simulink model "ACC_Model"  (Simulink 7.6)
settings: Solver=ode5  StartTime=0.0  StopTime=inf  FixedStep=1/100  RelTol=1e-3
undefined symbols (not defined in the file or in its folder): DiscIntNeverNeededParam
libraries: simulink x21, simulink_extras x6
(part 2 of 4)

== system ACC_Model/ACC_System/TIS2 Straight Road ==
  note: === TIS2 Straight Road block ===
      |
      |  - interpretes information provided from the second TIS sensor,
      |  - computes HeadWay Time (HWT) for object on the lane in front of the EGO car,
      |  - determines if detected objects is potentially dengerous,
      |  - outputs distance to the following car, computes its velocity and safe distance to be kept.
  EGO_velocity [m/s] : Inport
  TIS2_range [m] : Inport  Port=2  PortDimensions=TISdet(2)
  TIS2_rangedot [m/s] : Inport  Port=3  PortDimensions=TISdet(2)
  TIS2_theta [deg] : Inport  Port=4  PortDimensions=TISdet(2)
  HWT_dem [s] : Inport  Port=5
  Standstill [m] : Inport  Port=6
  HWT_dem [s]1 : InportShadow  Port=5
  Hold : Subsystem
  TIS2 Closest Object : Subsystem
  TIS2 HWT Computing : Subsystem
  TIS2 HWT Computing2 : Subsystem
  TIS2 HWT Flag : Subsystem
  TIS2 Lead Car Longitudinal Velocity : Subsystem
  TIS2 Objects On Lane : Subsystem
  TIS2 Sorting Fun : Subsystem
  TIS2_closest_object_search : Stateflow chart  TreatAsAtomicUnit=on
  HWT_flag : Outport
  TIS2 Lead distance [m] : Outport  Port=2
  TIS2 Safe_distance [m] : Outport  Port=3
  TIS2_HWT_straight : Outport  Port=4
  TIS2 Lead velocity [m/s] : Outport  Port=5
  index : Outport  Port=6
  wires:
  TIS2 Lead Car Longitudinal Velocity/1(Safe distance [m]) -> TIS2 Safe_distance [m]/1
  HWT_dem [s]/1 -> TIS2 Lead Car Longitudinal Velocity/1(HWT_dem (s)), TIS2 HWT Flag/2(HWT_dem [s])
  TIS2 Closest Object/1(rangedot [m/s]) -> TIS2 Lead Car Longitudinal Velocity/2(TIS2 Rangedot [m/s])
  TIS2 Closest Object/2(distance [m/s]) -> TIS2 Lead distance [m]/1, TIS2 HWT Computing2/1(Distance [m]), TIS2 HWT Flag/1(Distance closest [m])
  EGO_velocity [m/s]/1 -> TIS2 Lead Car Longitudinal Velocity/3(EGO Velocity [m/s]), TIS2 HWT Computing2/2(Velocity [m/s]), TIS2 HWT Computing/3(Velocity [m/s])
  TIS2 HWT Computing/1(HWT [s]) -> TIS2 HWT Flag/3(HWT [s])
  TIS2_closest_object_search/1(index) -> TIS2 Closest Object/3(index), index/1
  TIS2 Sorting Fun/3(TIS2_THETA [rad]) -> TIS2 Objects On Lane/3(TIS2_theta [rad])
  TIS2 Sorting Fun/2(TIS2_RANGEDOT [m/s]) -> TIS2 Objects On Lane/2(TIS2_rangedot [m/s])
  TIS2 Sorting Fun/1(TIS2_RANGE [m]) -> TIS2 Objects On Lane/1(TIS2_range [m])
  TIS2_theta [deg]/1 -> TIS2 Sorting Fun/3(TIS2theta [deg])
  TIS2_rangedot [m/s]/1 -> TIS2 Sorting Fun/2(TIS2rangedot [m/s])
  TIS2_range [m]/1 -> TIS2 Sorting Fun/1(TIS2range [m])
  Standstill [m]/1 -> TIS2 Lead Car Longitudinal Velocity/4(Standstill [m]), TIS2 HWT Flag/4(Standstill distance)
  TIS2 Objects On Lane/1(TIS2_RANGEDOT [m/s]) -> TIS2 Closest Object/1(TIS2_rangedot [m/s])
  TIS2 Lead Car Longitudinal Velocity/2(Lead velocity [m/s]) -> TIS2 Lead velocity [m/s]/1, Hold/2(lead_vel_in)
  TIS2 HWT Computing2/1(HWT [s]) -> TIS2_HWT_straight/1
  TIS2 HWT Flag/1(HWT_flag) -> Hold/1(HWTflagIN)
  Hold/1(HWT_flag) -> HWT_flag/1
  HWT_dem [s]1/1 -> TIS2 HWT Computing/2(HWT demanded)
  TIS2 Objects On Lane/2(TIS2_Distance [m]) -> TIS2 Closest Object/2(TIS2_distance [m]), TIS2_closest_object_search/1(distance), TIS2 HWT Computing/1(Distance [m])

== system ACC_Model/ACC_System/Display/If Action Subsystem ==
  note: === Display Module ===
      |
      |  - calls a GUI, which is updated at each step time,
      |  - Inputs for 'DISPLAY' block (msfcn_PlotSpeed):
      |    1 - RPM
      |    2 - EGO Velocity [kph]
      |    3 - Brake Pressure [bar]
      |    4 - Throttle [%]
      |    5 - ACC Flag
      |    6 - HWT converted
      |    7 - Lead car velocity [m/s]
      |
      |  - Output from DISPLAY block (msfcn_ACC_PlotSpeed function):
      |    1 - ACC system manual switch {0 - system off, 1 - system on}
  RPM1 : Inport
  EGO Velocity [m/s]1 : Inport  Port=2
  Brake_Pressure_[bar]1 : Inport  Port=3
  HWT_%1 : Inport  Port=4
  ACC_flag1 : Inport  Port=5
  Lead_car_velocity_[m/s]1 : Inport  Port=6
  Throttle_[%]1 : Inport  Port=7
  Action Port : ActionPort  PropagateVarSize=During execution  ActionType=then
  Brake Pressure [bar] : Gain  Gain=100/BrakePressureMax
  Brake Pressure [bar]1 : Gain  Gain=3.6
  DISPLAY : M-S-Function  FunctionName=msfcn_ACC_PlotSpeed  Parameters=DisplayFreq DisplaySwitch
      mask Display:
      | port_label('input',1,'RPM');
      | port_label('input',2,'EGO Velocity [km/h]');
      | port_label('input',3,'Brake Pressure [bar]');
      | port_label('input',4,'Throttle [%]');
      | port_label('input',5,'ACC Flag');
      | port_label('input',6,'HWT/HWT_dem-1 [%]');
      | port_label('input',7,'Lead car velocity [m/s]');
      | 
      | port_label('output',1,'System On/Off');
  Gain : Gain  OutDataTypeStr=double
  Rounding Function{,1..4,6} (6 alike) : Rounding  Operator=round
  m/s_kph1 : Gain  Gain=3.6
  "GUI_System ON {1} / OFF {0}1" : Outport  InitialOutput=1
  wires:
  Rounding Function/1 -> DISPLAY/1
  Rounding Function1/1 -> DISPLAY/2
  Rounding Function2/1 -> DISPLAY/3
  Rounding Function3/1 -> DISPLAY/4
  Brake Pressure [bar]/1 -> Rounding Function2/1
  Brake_Pressure_[bar]1/1 -> Brake Pressure [bar]/1
  Throttle_[%]1/1 -> Rounding Function3/1
  RPM1/1 -> Rounding Function/1
  m/s_kph1/1 -> Rounding Function4/1
  Rounding Function4/1 -> DISPLAY/7
  Rounding Function6/1 -> DISPLAY/5
  Gain/1 -> Rounding Function6/1
  EGO Velocity [m/s]1/1 -> Brake Pressure [bar]1/1
  ACC_flag1/1 -> Gain/1
  Lead_car_velocity_[m/s]1/1 -> m/s_kph1/1
  DISPLAY/1 -> "GUI_System ON {1} / OFF {0}1"/1
  HWT_%1/1 -> DISPLAY/6
  Brake Pressure [bar]1/1 -> Rounding Function1/1

== system ACC_Model/ACC_System/Display/If Action Subsystem1 ==
  Action Port : ActionPort  PropagateVarSize=During execution  ActionType=else
  Constant : Constant
  Out1 : Outport  InitialOutput=1
  wires:
  Constant/1 -> Out1/1

== system ACC_Model/ACC_System/Limitations1/cond ==
  In1 : Inport
  Integer Delay : simulink/Discrete/Integer Delay  NumDelays=1/Tsensor  InputProcessing=Inherited  vinit=0.0  samptime=Tsensor
  Logical Operator2 : Logic  Operator=NOT  AllPortsSameDT=off  OutDataTypeStr=boolean
  Logical Operator3 : Logic  Operator=OR  AllPortsSameDT=off  OutDataTypeStr=boolean
  Out1 : Outport
  wires:
  Logical Operator2/1 -> Logical Operator3/1, Integer Delay/1
  Integer Delay/1 -> Logical Operator3/2
  In1/1 -> Logical Operator2/1
  Logical Operator3/1 -> Out1/1

== system ACC_Model/ACC_System/Limitations2/cond1 ==
  In1 : Inport
  Integer Delay : simulink/Discrete/Integer Delay  NumDelays=1/Tsensor  InputProcessing=Inherited  vinit=0.0  samptime=Tsensor
  Logical Operator3 : Logic  Operator=OR  AllPortsSameDT=off  OutDataTypeStr=boolean
  Out1 : Outport
  wires:
  Integer Delay/1 -> Logical Operator3/2
  In1/1 -> Logical Operator3/1, Integer Delay/1
  Logical Operator3/1 -> Out1/1

== system ACC_Model/ACC_System/Radar/Radar ==
  TIS1 Range : Inport
  TIS1 Theta : Inport  Port=2
  TIS2 Range : Inport  Port=3
  TIS2 Theta : Inport  Port=4
  TIS1_index : Inport  Port=5
  TIS2_index : Inport  Port=6
  TIS1_HWT_% : Inport  Port=7
  TIS2_HWT_% : Inport  Port=8
  System switch : Inport  Port=9
  Enable : EnablePort  PropagateVarSize=During execution
  Level-2 M-file S-Function : M-S-Function  FunctionName=msfcn_ACC_radar_graph  Parameters=RadarFreq TISdet TISMaxRange TISMaxTheta RadarSwitch
  Logical Operator : Logic  AllPortsSameDT=off  OutDataTypeStr=boolean
  Logical Operator1 : Logic  AllPortsSameDT=off  OutDataTypeStr=boolean
  Product1 : Product  RndMeth=Zero
  Product2 : Product  RndMeth=Zero
  wires:
  TIS1 Range/1 -> Level-2 M-file S-Function/1
  TIS1 Theta/1 -> Level-2 M-file S-Function/2
  TIS2 Range/1 -> Level-2 M-file S-Function/3
  TIS2 Theta/1 -> Level-2 M-file S-Function/4
  TIS1_HWT_%/1 -> Logical Operator/1
  TIS2_HWT_%/1 -> Logical Operator1/1
  Logical Operator/1 -> Level-2 M-file S-Function/7
  Logical Operator1/1 -> Level-2 M-file S-Function/8
  System switch/1 -> Logical Operator1/2, Logical Operator/2, Product2/2, Product1/2
  Product2/1 -> Level-2 M-file S-Function/6
  Product1/1 -> Level-2 M-file S-Function/5
  TIS1_index/1 -> Product1/1
  TIS2_index/1 -> Product2/1

== system ACC_Model/ACC_System/TIS1 ACC action/If Action Subsystem ==
  rd : Inport
  e : Inport  Port=2
  Vp : Inport  Port=3
  EGO distance : Inport  Port=4
  HWT dem : Inport  Port=5
  th in : Inport  Port=6
  Action Port : ActionPort  PropagateVarSize=During execution  ActionType=then
  If : If  IfExpression=u1 <= 0  SampleTime=Tsensor
  If Action Subsystem : Subsystem  TreatAsAtomicUnit=on
  If Action Subsystem1 : Subsystem  TreatAsAtomicUnit=on
  Merge : Merge
  Merge1 : Merge
  Rate Limiter : RateLimiter  RisingSlewLimit=BrakeMax*1e3  FallingSlewLimit=-BrakeMax*1e3  SampleTimeMode=inherited
  e1 : InportShadow  Port=2
  th in1 : InportShadow  Port=6
  dec : Outport  InitialOutput=0
  throttle : Outport  Port=2  InitialOutput=0
  wires:
  rd/1 -> If/1, If Action Subsystem1/1(rd)
  If/1 -> If Action Subsystem/Action
  If/2 -> If Action Subsystem1/Action
  e/1 -> If Action Subsystem/1(e)
  If Action Subsystem/1(brake) -> Merge/1
  If Action Subsystem1/1(dec) -> Merge/2
  If Action Subsystem/2(throttle) -> Merge1/1
  If Action Subsystem1/2(throttle) -> Merge1/2
  Merge/1 -> dec/1
  Merge1/1 -> Rate Limiter/1
  Vp/1 -> If Action Subsystem1/3(Vp)
  e1/1 -> If Action Subsystem1/2(e)
  EGO distance/1 -> If Action Subsystem1/4(EGO distance)
  HWT dem/1 -> If Action Subsystem1/5(HWT_dem)
  th in/1 -> If Action Subsystem/2(th_in)
  th in1/1 -> If Action Subsystem1/6(th_in)
  Rate Limiter/1 -> throttle/1

== system ACC_Model/ACC_System/TIS1 ACC action/If Action Subsystem1 ==
  rd : Inport
  e : Inport  Port=2
  Vp : Inport  Port=3
  EGO dis : Inport  Port=4
  HWT dem : Inport  Port=5
  Action Port : ActionPort  PropagateVarSize=During execution  ActionType=else
  If : If  IfExpression=u1 <= 0  SampleTime=Tsensor
  If Action Subsystem : Subsystem  TreatAsAtomicUnit=on
  If Action Subsystem1 : Subsystem  TreatAsAtomicUnit=on
  Merge : Merge
  Merge1 : Merge
  dec : Outport  InitialOutput=0
  throttle : Outport  Port=2  InitialOutput=0
  wires:
  rd/1 -> If/1, If Action Subsystem1/1(rd)
  If/1 -> If Action Subsystem/Action
  If/2 -> If Action Subsystem1/Action
  Vp/1 -> If Action Subsystem1/3(Vp)
  If Action Subsystem/1(dec) -> Merge/1
  If Action Subsystem1/2(throttle) -> Merge1/2
  Merge/1 -> dec/1
  Merge1/1 -> throttle/1
  If Action Subsystem1/1(dec) -> Merge/2
  If Action Subsystem/2(throttle) -> Merge1/1
  e/1 -> If Action Subsystem1/2(e)
  EGO dis/1 -> If Action Subsystem1/4(Ego distance)
  HWT dem/1 -> If Action Subsystem1/5(HWT dem)

== system ACC_Model/ACC_System/TIS1 Bend Road/Hold ==
  HWTflagIN : Inport
  lead_vel_in : Inport  Port=2
  HWTflagIN1 : InportShadow  Port=1
  If : If  IfExpression=u1 < 0.1  SampleTime=Tsensor
  If Action Subsystem : Subsystem  TreatAsAtomicUnit=on
  If Action Subsystem1 : Subsystem  TreatAsAtomicUnit=on
  Merge : Merge
  HWT_flag : Outport
  wires:
  lead_vel_in/1 -> If/1
  If/1 -> If Action Subsystem/Action
  If/2 -> If Action Subsystem1/Action
  If Action Subsystem/1(Out1) -> Merge/1
  If Action Subsystem1/1(Out1) -> Merge/2
  Merge/1 -> HWT_flag/1
  HWTflagIN/1 -> If Action Subsystem1/1(In1)
  HWTflagIN1/1 -> If Action Subsystem/1(In1)

== system ACC_Model/ACC_System/TIS1 Bend Road/Lead Car Longitudinal Velocity ==
  note: === TIS1 Lead Car Longitudinal Velocity block ===
      |
      |  - computes the leading car absolute velocity and safe distance between the EGO and leading car.
  HWT_dem (s) : Inport
  TIS1 Rangedot [m/s] : Inport  Port=2
  EGO Velocity [m/s] : Inport  Port=3
  Standstill [m] : Inport  Port=4
  theta [rad] : Inport  Port=5
  lambda [rad] : Inport  Port=6
  TIS1 Range [m] : Inport  Port=7
  Abs : Abs
  Add : Sum  Inputs=+-  RndMeth=Zero
  Add1 : Sum  Inputs=+-
  Constant : Constant  Value=0
  Divide : Product  Inputs=*/
  Divide2 : Product  Inputs=*/
  HWT_dem (s)1 : InportShadow  Port=1
  Product : Product  RndMeth=Zero
  Relational Operator : RelationalOperator  Operator=<=  OutDataTypeStr=boolean
  Switch : Switch  Criteria=u2 > Threshold
  Switch1 : Switch  Threshold=TISMaxRange(1)
  Trigonometric Function : Trigonometry  Operator=cos
  Safe distance [m] : Outport
  Lead velocity [m/s] : Outport  Port=2
  wires:
  Relational Operator/1 -> Switch/2
  Divide/1 -> Relational Operator/2
  HWT_dem (s)1/1 -> Divide/2
  Standstill [m]/1 -> Switch/1, Divide/1
  Switch/1 -> Safe distance [m]/1
  Product/1 -> Switch/3
  HWT_dem (s)/1 -> Product/2
  Add/1 -> Abs/1
  TIS1 Rangedot [m/s]/1 -> Divide2/1
  EGO Velocity [m/s]/1 -> Add/1
  lambda [rad]/1 -> Add1/1
  theta [rad]/1 -> Add1/2
  Add1/1 -> Trigonometric Function/1
  Trigonometric Function/1 -> Divide2/2
  Divide2/1 -> Add/2
  Abs/1 -> Product/1, Relational Operator/1, Switch1/3
  TIS1 Range [m]/1 -> Switch1/2
  Constant/1 -> Switch1/1
  Switch1/1 -> Lead velocity [m/s]/1

== system ACC_Model/ACC_System/TIS1 Bend Road/TIS1 Closest Object On Bend Road ==
  note: === TIS1 Closest Object block ===
      |
      |  - passing through data about potentially the most dangerous object driving on the bend road.
  index : Inport
  TIS1_range [m] : Inport  Port=2
  TIS1_rangedot [m] : Inport  Port=3
  TIS1_theta [rad] : Inport  Port=4
  TIS1_Distance [m] : Inport  Port=5
  TIS1_lambda [rad] : Inport  Port=6
  Constant2 : Constant  Value=TISMaxRange(1)
  Selector{1..3,6..7} (5 alike) : Selector  InputPortWidth=TISdet(1)  IndexOptions=Index vector (port)  Indices=[1 3]  OutputSizes=1
  Switch : Switch  Criteria=u2 ~= 0
  range [m] : Outport
  rangedot [m/s] : Outport  Port=2
  theta [rad] : Outport  Port=3
  Distance [m] : Outport  Port=4
  lambda [rad] : Outport  Port=5
  wires:
  TIS1_rangedot [m]/1 -> Selector2/1
  TIS1_range [m]/1 -> Selector1/1
  index/1 -> Selector1/2, Selector2/2, Selector3/2, Selector6/2, Selector7/2
  TIS1_theta [rad]/1 -> Selector3/1
  TIS1_Distance [m]/1 -> Selector6/1
  TIS1_lambda [rad]/1 -> Selector7/1
  Selector1/1 -> range [m]/1
  Selector2/1 -> rangedot [m/s]/1
  Selector3/1 -> theta [rad]/1
  Selector7/1 -> lambda [rad]/1
  Selector6/1 -> Switch/2, Switch/1
  Constant2/1 -> Switch/3
  Switch/1 -> Distance [m]/1

== system ACC_Model/ACC_System/TIS1 Bend Road/TIS1 HWT Computing ==
  note: === TIS1 HWT Computing block===
      |
      |  - computes HeadWay Time (HWT) as it is defined in ISO norms.
  Distance [m] : Inport
  Velocity [m/s] : Inport  Port=2
  If : If
  If Action Subsystem : Subsystem  TreatAsAtomicUnit=on
  If Action Subsystem1 : Subsystem  TreatAsAtomicUnit=on
  Merge : Merge
  HWT [s] : Outport
  wires:
  Velocity [m/s]/1 -> If/1, If Action Subsystem/2(Velocity [m/s])
  If/1 -> If Action Subsystem/Action
  If/2 -> If Action Subsystem1/Action
  If Action Subsystem/1(HWT [s]) -> Merge/1
  If Action Subsystem1/1(Out1) -> Merge/2
  Merge/1 -> HWT [s]/1
  Distance [m]/1 -> If Action Subsystem/1(Distance [m])

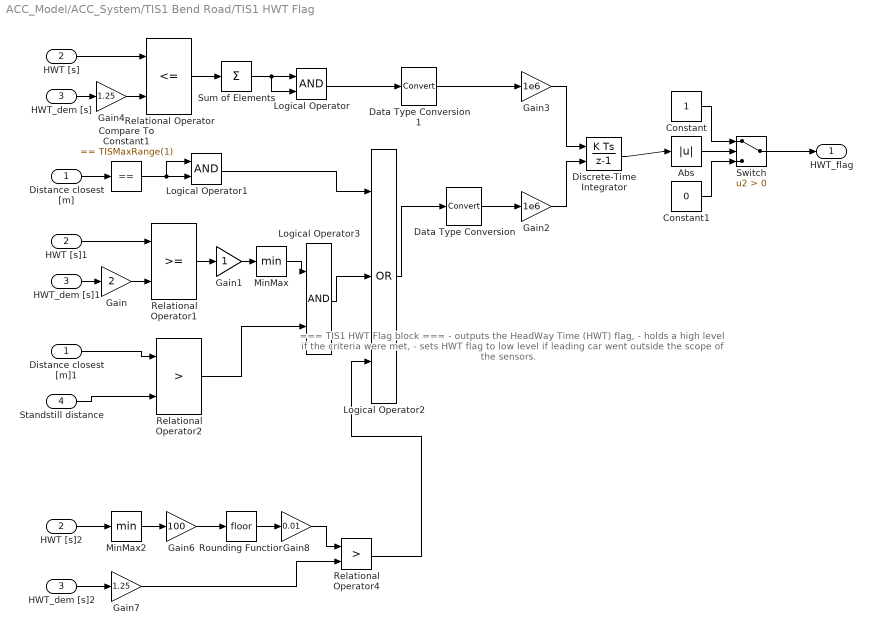
== system ACC_Model/ACC_System/TIS1 Bend Road/TIS1 HWT Flag ==
  note: === TIS1 HWT Flag block ===
      |
      |  - outputs the HeadWay Time (HWT) flag,
      |  - holds a high level if the criteria were met,
      |  - sets HWT flag to low level if leading car
      |    went outside the scope of the sensors.
  Distance closest [m] : Inport
  HWT [s] : Inport  Port=2
  HWT_dem [s] : Inport  Port=3
  Standstill distance : Inport  Port=4
  Abs : Abs
  Compare To Constant1 : simulink/Logic and Bit Operations/Compare To Constant  SystemSampleTime=-1  relop===  const=TISMaxRange(1)  LogicOutDataTypeMode=uint8
  Constant : Constant
  Constant1 : Constant  Value=0
  Data Type Conversion : DataTypeConversion
  Data Type Conversion1 : DataTypeConversion
  Discrete-Time Integrator : DiscreteIntegrator  ExternalReset=level  SampleTime=Tsensor  ICPrevOutput=DiscIntNeverNeededParam  ICPrevScaledInput=DiscIntNeverNeededParam
  Distance closest [m]1 : InportShadow  Port=1
  Gain : Gain  Gain=2
  Gain1 : Gain
  Gain2 : Gain  Gain=1e6  OutDataTypeStr=double
  Gain3 : Gain  Gain=1e6  OutDataTypeStr=double
  Gain4 : Gain  Gain=1.25
  Gain6 : Gain  Gain=100
  Gain7 : Gain  Gain=1.25
  Gain8 : Gain  Gain=0.01
  HWT [s]1 : InportShadow  Port=2
  HWT [s]2 : InportShadow  Port=2
  HWT_dem [s]1 : InportShadow  Port=3
  HWT_dem [s]2 : InportShadow  Port=3
  Logical Operator : Logic  AllPortsSameDT=off  OutDataTypeStr=boolean
  Logical Operator1 : Logic  AllPortsSameDT=off  OutDataTypeStr=boolean
  Logical Operator2 : Logic  Operator=OR  Inputs=3  AllPortsSameDT=off  OutDataTypeStr=boolean
  Logical Operator3 : Logic  AllPortsSameDT=off  OutDataTypeStr=boolean
  MinMax : MinMax
  MinMax2 : MinMax
  Relational Operator : RelationalOperator  Operator=<=  OutDataTypeStr=boolean
  Relational Operator1 : RelationalOperator  OutDataTypeStr=boolean
  Relational Operator2 : RelationalOperator  Operator=>  OutDataTypeStr=boolean
  Relational Operator4 : RelationalOperator  Operator=>  OutDataTypeStr=boolean
  Rounding Function : Rounding
  Sum of Elements : Sum  Inputs=+
  Switch : Switch  Criteria=u2 > Threshold
  HWT_flag : Outport
  wires:
  Logical Operator1/1 -> Logical Operator2/1
  Distance closest [m]/1 -> Compare To Constant1/1
  Logical Operator/1 -> Data Type Conversion1/1
  Sum of Elements/1 -> Logical Operator/2, Logical Operator/1
  Relational Operator/1 -> Sum of Elements/1
  HWT_dem [s]/1 -> Gain4/1
  HWT [s]/1 -> Relational Operator/1
  Compare To Constant1/1 -> Logical Operator1/2, Logical Operator1/1
  HWT [s]1/1 -> Relational Operator1/1
  Gain/1 -> Relational Operator1/2
  Relational Operator1/1 -> Gain1/1
  Gain1/1 -> MinMax/1
  Logical Operator2/1 -> Data Type Conversion/1
  HWT_dem [s]1/1 -> Gain/1
  Distance closest [m]1/1 -> Relational Operator2/1
  Standstill distance/1 -> Relational Operator2/2
  Relational Operator2/1 -> Logical Operator3/2
  MinMax/1 -> Logical Operator3/1
  Logical Operator3/1 -> Logical Operator2/2
  Gain2/1 -> Discrete-Time Integrator/2
  Gain3/1 -> Discrete-Time Integrator/1
  Discrete-Time Integrator/1 -> Abs/1
  Abs/1 -> Switch/2
  Constant/1 -> Switch/1
  Constant1/1 -> Switch/3
  Switch/1 -> HWT_flag/1
  Gain4/1 -> Relational Operator/2
  Relational Operator4/1 -> Logical Operator2/3
  HWT_dem [s]2/1 -> Gain7/1
  HWT [s]2/1 -> MinMax2/1
  Gain6/1 -> Rounding Function/1
  Rounding Function/1 -> Gain8/1
  MinMax2/1 -> Gain6/1
  Gain8/1 -> Relational Operator4/1
  Gain7/1 -> Relational Operator4/2
  Data Type Conversion/1 -> Gain2/1
  Data Type Conversion1/1 -> Gain3/1

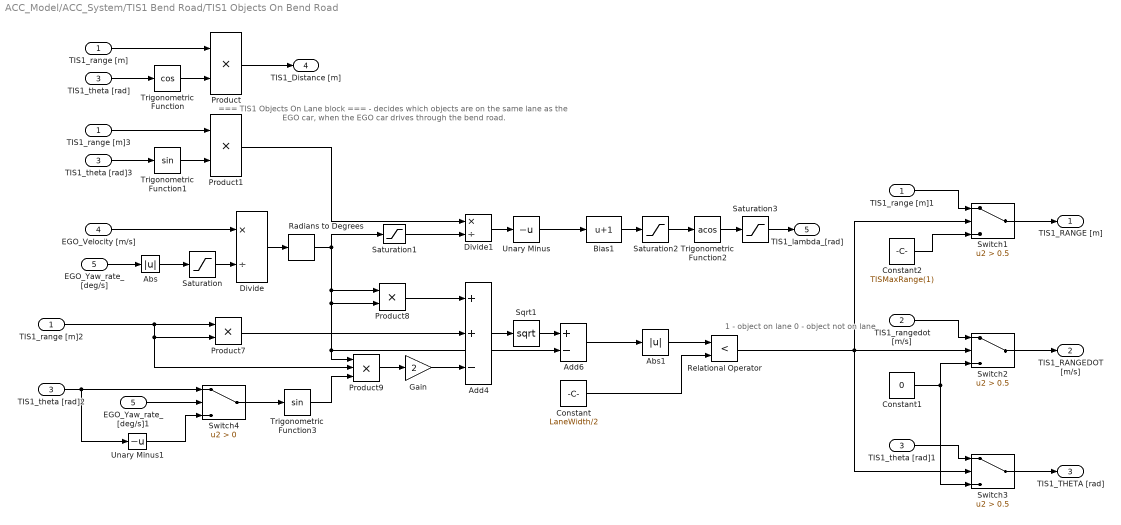
== system ACC_Model/ACC_System/TIS1 Bend Road/TIS1 Objects On Bend Road ==
  note: 1  - object      on lane
      | 0 - object not on lane
  note: === TIS1 Objects On Lane block ===
      |
      |  - decides which objects are on the same lane as the EGO car,
      |     when the EGO car drives through the bend road.
  TIS1_range [m] : Inport
  TIS1_rangedot [m/s] : Inport  Port=2
  TIS1_theta [rad] : Inport  Port=3
  EGO_Velocity [m/s] : Inport  Port=4
  EGO_Yaw_rate_[deg/s] : Inport  Port=5
  Abs : Abs
  Abs1 : Abs
  Add4 : Sum  Inputs=++-
  Add6 : Sum  Inputs=+-
  Bias1 : Bias  Bias=1
  Constant : Constant  Value=LaneWidth/2
  Constant1 : Constant  Value=0
  Constant2 : Constant  Value=TISMaxRange(1)
  Divide : Product  Inputs=*/
  Divide1 : Product  Inputs=*/
  EGO_Yaw_rate_[deg/s]1 : InportShadow  Port=5
  Gain : Gain  Gain=2
  Product{,1,7..8} (4 alike) : Product  RndMeth=Zero
  Product9 : Product  Inputs=3  RndMeth=Zero
  Radians to Degrees : simulink_extras/Transformations/Radians to Degrees  SystemSampleTime=-1
  Relational Operator : RelationalOperator  Operator=<  OutDataTypeStr=boolean
  Saturation : Saturate  UpperLimit=inf  LowerLimit=1e-6
  Saturation1 : Saturate  UpperLimit=inf  LowerLimit=1e-6
  Saturation2 : Saturate  UpperLimit=1  LowerLimit=-1
  Saturation3 : Saturate  UpperLimit=pi  LowerLimit=0
  Sqrt1 : Math  Operator=sqrt  SaturateOnIntegerOverflow=on
  Switch1 : Switch  Criteria=u2 > Threshold  Threshold=0.5
  Switch2 : Switch  Criteria=u2 > Threshold  Threshold=0.5
  Switch3 : Switch  Criteria=u2 > Threshold  Threshold=0.5
  Switch4 : Switch  Criteria=u2 > Threshold
  TIS1_range [m]1 : InportShadow  Port=1
  TIS1_range [m]2 : InportShadow  Port=1
  TIS1_range [m]3 : InportShadow  Port=1
  TIS1_theta [rad]1 : InportShadow  Port=3
  TIS1_theta [rad]2 : InportShadow  Port=3
  TIS1_theta [rad]3 : InportShadow  Port=3
  Trigonometric Function : Trigonometry  Operator=cos
  Trigonometric Function1 : Trigonometry
  Trigonometric Function2 : Trigonometry  Operator=acos
  Trigonometric Function3 : Trigonometry
  Unary Minus : UnaryMinus
  Unary Minus1 : UnaryMinus
  TIS1_RANGE [m] : Outport
  TIS1_RANGEDOT [m/s] : Outport  Port=2
  TIS1_THETA [rad] : Outport  Port=3
  TIS1_Distance [m] : Outport  Port=4
  TIS1_lambda_[rad] : Outport  Port=5
  wires:
  TIS1_range [m]/1 -> Product/1
  TIS1_theta [rad]/1 -> Trigonometric Function/1
  Trigonometric Function/1 -> Product/2
  Trigonometric Function1/1 -> Product1/2
  EGO_Velocity [m/s]/1 -> Divide/1
  EGO_Yaw_rate_[deg/s]/1 -> Abs/1
  Divide/1 -> Radians to Degrees/1
  Radians to Degrees/1 -> Product8/1, Product8/2, Product9/1, Add6/2, Saturation1/1
  Relational Operator/1 -> Switch1/2, Switch2/2, Switch3/2
  TIS1_rangedot [m/s]/1 -> Switch2/1
  TIS1_range [m]1/1 -> Switch1/1
  TIS1_theta [rad]1/1 -> Switch3/1
  Constant1/1 -> Switch2/3, Switch3/3
  Constant2/1 -> Switch1/3
  Switch1/1 -> TIS1_RANGE [m]/1
  Switch2/1 -> TIS1_RANGEDOT [m/s]/1
  Switch3/1 -> TIS1_THETA [rad]/1
  Bias1/1 -> Saturation2/1
  Divide1/1 -> Unary Minus/1
  Unary Minus/1 -> Bias1/1
  Trigonometric Function2/1 -> Saturation3/1
  Product/1 -> TIS1_Distance [m]/1
  Product8/1 -> Add4/1
  Product7/1 -> Add4/2
  Gain/1 -> Add4/3
  Product9/1 -> Gain/1
  Trigonometric Function3/1 -> Product9/3
  Add4/1 -> Sqrt1/1
  Sqrt1/1 -> Add6/1
  Add6/1 -> Abs1/1
  EGO_Yaw_rate_[deg/s]1/1 -> Switch4/2
  Switch4/1 -> Trigonometric Function3/1
  TIS1_theta [rad]2/1 -> Switch4/1, Unary Minus1/1
  Unary Minus1/1 -> Switch4/3
  TIS1_range [m]2/1 -> Product7/1, Product7/2, Product9/2
  TIS1_range [m]3/1 -> Product1/1
  TIS1_theta [rad]3/1 -> Trigonometric Function1/1
  Product1/1 -> Divide1/1
  Abs1/1 -> Relational Operator/1
  Constant/1 -> Relational Operator/2
  Saturation/1 -> Divide/2
  Saturation1/1 -> Divide1/2
  Saturation2/1 -> Trigonometric Function2/1
  Saturation3/1 -> TIS1_lambda_[rad]/1
  Abs/1 -> Saturation/1

== system ACC_Model/ACC_System/TIS1 Bend Road/TIS1 Sorting  Fun ==
  note: === TIS1 Sorting Fun block ===
      |
      |  - transforms information from the first sensor
      |    to the more appropriate form.
  TIS1range [m] : Inport
  TIS1rangedot [m/s] : Inport  Port=2
  TIS1theta [deg] : Inport  Port=3
  Degrees to Radians : simulink_extras/Transformations/Degrees to Radians  SystemSampleTime=-1
  Switch : Switch  Criteria=u2 ~= 0
  Unary Minus : UnaryMinus
  Unary Minus1 : UnaryMinus
  range max : Constant  Value=TISMaxRange(1)
  TIS1_RANGE [m] : Outport
  TIS1_RANGEDOT [m/s] : Outport  Port=2
  TIS1_THETA [rad] : Outport  Port=3
  wires:
  Unary Minus1/1 -> TIS1_RANGEDOT [m/s]/1
  TIS1theta [deg]/1 -> Unary Minus/1
  TIS1range [m]/1 -> Switch/2, Switch/1
  Degrees to Radians/1 -> TIS1_THETA [rad]/1
  range max/1 -> Switch/3
  TIS1rangedot [m/s]/1 -> Unary Minus1/1
  Switch/1 -> TIS1_RANGE [m]/1
  Unary Minus/1 -> Degrees to Radians/1

== system ACC_Model/ACC_System/TIS1 Straight Road/Hold ==
  HWTflagIN : Inport
  lead_vel_in : Inport  Port=2
  HWTflagIN1 : InportShadow  Port=1
  If : If  IfExpression=u1 < 0.1  SampleTime=Tsensor
  If Action Subsystem : Subsystem  TreatAsAtomicUnit=on
  If Action Subsystem1 : Subsystem  TreatAsAtomicUnit=on
  Merge : Merge
  HWT_flag : Outport
  wires:
  lead_vel_in/1 -> If/1
  If/1 -> If Action Subsystem/Action
  If/2 -> If Action Subsystem1/Action
  If Action Subsystem/1(Out1) -> Merge/1
  If Action Subsystem1/1(Out1) -> Merge/2
  Merge/1 -> HWT_flag/1
  HWTflagIN/1 -> If Action Subsystem1/1(In1)
  HWTflagIN1/1 -> If Action Subsystem/1(In1)

== system ACC_Model/ACC_System/TIS1 Straight Road/TIS1 Closest Object ==
  note: === TIS1 Closest Object block ===
      |
      |  - passing through data about potentially the most dangerous object driving on the straight road.
  TIS1_rangedot [m/s] : Inport
  TIS1_Distance [m] : Inport  Port=2
  index : Inport  Port=3
  Selector1 : Selector  InputPortWidth=TISdet(1)  IndexOptions=Index vector (port)  Indices=[1 3]  OutputSizes=1
  Selector2 : Selector  InputPortWidth=TISdet(1)  IndexOptions=Index vector (port)  Indices=[1 3]  OutputSizes=1
  rangedot [m/s] : Outport
  Distance [m/s] : Outport  Port=2
  wires:
  index/1 -> Selector1/2, Selector2/2
  TIS1_rangedot [m/s]/1 -> Selector1/1
  Selector1/1 -> rangedot [m/s]/1
  TIS1_Distance [m]/1 -> Selector2/1
  Selector2/1 -> Distance [m/s]/1

== system ACC_Model/ACC_System/TIS1 Straight Road/TIS1 HWT Computing ==
  note: === TIS1 HWT Computing block===
      |
      |  - computes HeadWay Time (HWT) as it is defined in ISO norms.
  Distance [m] : Inport
  HWT demanded : Inport  Port=2
  Velocity [m/s] : Inport  Port=3
  If : If
  If Action Subsystem : Subsystem  TreatAsAtomicUnit=on
  If Action Subsystem1 : Subsystem  TreatAsAtomicUnit=on
  Merge : Merge
  HWT [s] : Outport
  wires:
  Velocity [m/s]/1 -> If/1, If Action Subsystem/2(Velocity [m/s])
  If/1 -> If Action Subsystem/Action
  If/2 -> If Action Subsystem1/Action
  If Action Subsystem/1(HWT [s]) -> Merge/1
  If Action Subsystem1/1(Out1) -> Merge/2
  Merge/1 -> HWT [s]/1
  Distance [m]/1 -> If Action Subsystem/1(Distance [m])
  HWT demanded/1 -> If Action Subsystem1/1(HWT demanded [s])

== system ACC_Model/ACC_System/TIS1 Straight Road/TIS1 HWT Computing1 ==
  note: === TIS1 HWT Computing block===
      |
      |  - computes HeadWay Time (HWT) as it is defined in ISO norms.
  Distance [m] : Inport
  Velocity [m/s] : Inport  Port=2
  If : If
  If Action Subsystem : Subsystem  TreatAsAtomicUnit=on
  If Action Subsystem1 : Subsystem  TreatAsAtomicUnit=on
  Merge : Merge
  HWT [s] : Outport
  wires:
  Velocity [m/s]/1 -> If/1, If Action Subsystem/2(Velocity [m/s])
  If/1 -> If Action Subsystem/Action
  If/2 -> If Action Subsystem1/Action
  If Action Subsystem/1(HWT [s]) -> Merge/1
  If Action Subsystem1/1(Out1) -> Merge/2
  Merge/1 -> HWT [s]/1
  Distance [m]/1 -> If Action Subsystem/1(Distance [m])

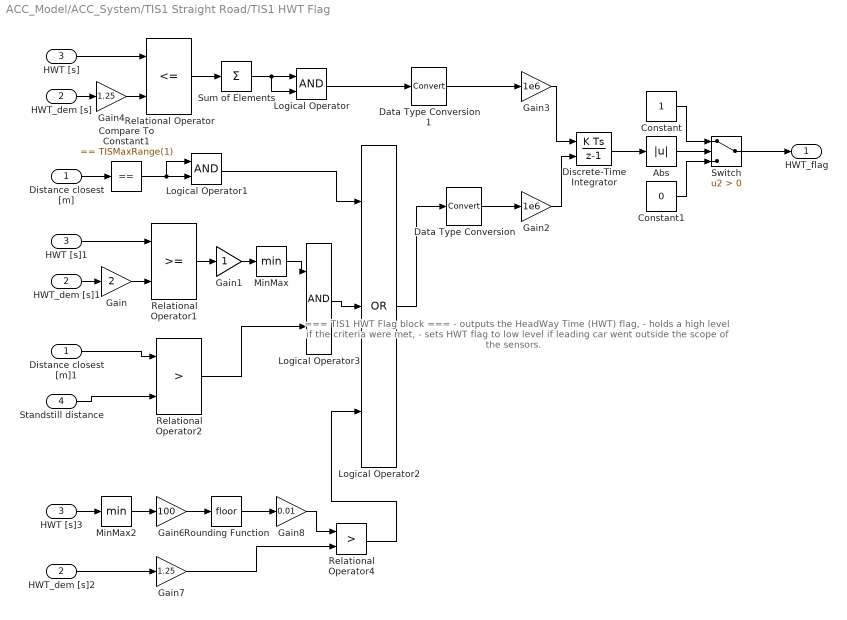
== system ACC_Model/ACC_System/TIS1 Straight Road/TIS1 HWT Flag ==
  note: === TIS1 HWT Flag block ===
      |
      |  - outputs the HeadWay Time (HWT) flag,
      |  - holds a high level if the criteria were met,
      |  - sets HWT flag to low level if leading car
      |    went outside the scope of the sensors.
  Distance closest [m] : Inport
  HWT_dem [s] : Inport  Port=2
  HWT [s] : Inport  Port=3
  Standstill distance : Inport  Port=4
  Abs : Abs
  Compare To Constant1 : simulink/Logic and Bit Operations/Compare To Constant  SystemSampleTime=-1  relop===  const=TISMaxRange(1)  LogicOutDataTypeMode=uint8
  Constant : Constant
  Constant1 : Constant  Value=0
  Data Type Conversion : DataTypeConversion
  Data Type Conversion1 : DataTypeConversion
  Discrete-Time Integrator : DiscreteIntegrator  ExternalReset=level  SampleTime=Tsensor  ICPrevOutput=DiscIntNeverNeededParam  ICPrevScaledInput=DiscIntNeverNeededParam
  Distance closest [m]1 : InportShadow  Port=1
  Gain : Gain  Gain=2
  Gain1 : Gain
  Gain2 : Gain  Gain=1e6  OutDataTypeStr=double
  Gain3 : Gain  Gain=1e6  OutDataTypeStr=double
  Gain4 : Gain  Gain=1.25
  Gain6 : Gain  Gain=100
  Gain7 : Gain  Gain=1.25
  Gain8 : Gain  Gain=0.01
  HWT [s]1 : InportShadow  Port=3
  HWT [s]3 : InportShadow  Port=3
  HWT_dem [s]1 : InportShadow  Port=2
  HWT_dem [s]2 : InportShadow  Port=2
  Logical Operator : Logic  AllPortsSameDT=off  OutDataTypeStr=boolean
  Logical Operator1 : Logic  AllPortsSameDT=off  OutDataTypeStr=boolean
  Logical Operator2 : Logic  Operator=OR  Inputs=3  AllPortsSameDT=off  OutDataTypeStr=boolean
  Logical Operator3 : Logic  AllPortsSameDT=off  OutDataTypeStr=boolean
  MinMax : MinMax
  MinMax2 : MinMax
  Relational Operator : RelationalOperator  Operator=<=  OutDataTypeStr=boolean
  Relational Operator1 : RelationalOperator  OutDataTypeStr=boolean
  Relational Operator2 : RelationalOperator  Operator=>  OutDataTypeStr=boolean
  Relational Operator4 : RelationalOperator  Operator=>  OutDataTypeStr=boolean
  Rounding Function : Rounding
  Sum of Elements : Sum  Inputs=+
  Switch : Switch  Criteria=u2 > Threshold
  HWT_flag : Outport
  wires:
  Logical Operator1/1 -> Logical Operator2/1
  Distance closest [m]/1 -> Compare To Constant1/1
  Logical Operator/1 -> Data Type Conversion1/1
  Sum of Elements/1 -> Logical Operator/2, Logical Operator/1
  Relational Operator/1 -> Sum of Elements/1
  HWT_dem [s]/1 -> Gain4/1
  HWT [s]/1 -> Relational Operator/1
  Compare To Constant1/1 -> Logical Operator1/2, Logical Operator1/1
  HWT [s]1/1 -> Relational Operator1/1
  Gain/1 -> Relational Operator1/2
  Relational Operator1/1 -> Gain1/1
  Gain1/1 -> MinMax/1
  Logical Operator2/1 -> Data Type Conversion/1
  HWT_dem [s]1/1 -> Gain/1
  Distance closest [m]1/1 -> Relational Operator2/1
  Standstill distance/1 -> Relational Operator2/2
  Relational Operator2/1 -> Logical Operator3/2
  MinMax/1 -> Logical Operator3/1
  Logical Operator3/1 -> Logical Operator2/2
  Gain2/1 -> Discrete-Time Integrator/2
  Gain3/1 -> Discrete-Time Integrator/1
  Discrete-Time Integrator/1 -> Abs/1
  Switch/1 -> HWT_flag/1
  Abs/1 -> Switch/2
  Constant/1 -> Switch/1
  Constant1/1 -> Switch/3
  Gain4/1 -> Relational Operator/2
  HWT_dem [s]2/1 -> Gain7/1
  HWT [s]3/1 -> MinMax2/1
  Gain6/1 -> Rounding Function/1
  Rounding Function/1 -> Gain8/1
  MinMax2/1 -> Gain6/1
  Gain8/1 -> Relational Operator4/1
  Gain7/1 -> Relational Operator4/2
  Relational Operator4/1 -> Logical Operator2/3
  Data Type Conversion/1 -> Gain2/1
  Data Type Conversion1/1 -> Gain3/1

== system ACC_Model/ACC_System/TIS1 Straight Road/TIS1 Lead Car Longitudinal Velocity ==
  note: === TIS1 Lead Car Longitudinal Velocity block ===
      |
      |  - computes the leading car absolute velocity and safe distance between the EGO and leading car.
  HWT_dem (s) : Inport
  TIS1 Rangedot [m/s] : Inport  Port=2
  EGO Velocity [m/s] : Inport  Port=3
  Standstill [m] : Inport  Port=4
  Abs : Abs
  Add : Sum  Inputs=+-
  Constant : Constant  Value=0
  Divide : Product  Inputs=*/
  HWT_dem (s)1 : InportShadow  Port=1
  Product : Product  RndMeth=Zero
  Relational Operator : RelationalOperator  Operator=<=  OutDataTypeStr=boolean
  Switch : Switch  Criteria=u2 > Threshold
  Switch1 : Switch  Criteria=u2 ~= 0
  TIS1 Rangedot [m/s]1 : InportShadow  Port=2
  lead_velocity [m/s] : Outport
  Safe distance [m] : Outport  Port=2
  wires:
  EGO Velocity [m/s]/1 -> Add/1
  TIS1 Rangedot [m/s]/1 -> Add/2
  Add/1 -> Abs/1
  HWT_dem (s)/1 -> Product/2
  Product/1 -> Switch/3
  Switch/1 -> Safe distance [m]/1
  Standstill [m]/1 -> Divide/1, Switch/1
  HWT_dem (s)1/1 -> Divide/2
  Divide/1 -> Relational Operator/2
  Relational Operator/1 -> Switch/2
  TIS1 Rangedot [m/s]1/1 -> Switch1/2
  Constant/1 -> Switch1/3
  Switch1/1 -> lead_velocity [m/s]/1
  Abs/1 -> Product/1, Relational Operator/1, Switch1/1

== system ACC_Model/ACC_System/TIS1 Straight Road/TIS1 Objects On Lane ==
  note: === TIS1 Objects On Lane block ===
      |
      |  - decides which objects are on the same lane as the EGO car,
      |    when the EGO car drives straight.
  TIS1_range [m] : Inport
  TIS1_rangedot [m/s] : Inport  Port=2
  TIS1_theta [rad] : Inport  Port=3
  Abs : Abs
  Compare To Constant : simulink/Logic and Bit Operations/Compare To Constant  SystemSampleTime=-1  relop=<  const=LaneWidth/2  LogicOutDataTypeMode=boolean
  Constant : Constant  Value=0
  Product : Product  RndMeth=Zero
  Product1 : Product  RndMeth=Zero
  Switch1 : Switch  Criteria=u2 > Threshold  Threshold=0.5
  Switch3 : Switch  Criteria=u2 > Threshold  Threshold=0.5
  TIS1 range max : Constant  Value=TISMaxRange(1)
  Trigonometric Function : Trigonometry
  Trigonometric Function1 : Trigonometry  Operator=cos
  TIS1_RANGEDOT [m/s] : Outport
  TIS1_Distance [m] : Outport  Port=2
  wires:
  TIS1_theta [rad]/1 -> Abs/1, Trigonometric Function1/1
  Trigonometric Function/1 -> Product/2
  Product/1 -> Compare To Constant/1
  TIS1_range [m]/1 -> Product/1, Product1/1
  TIS1_rangedot [m/s]/1 -> Switch1/1
  Switch1/1 -> TIS1_RANGEDOT [m/s]/1
  Switch3/1 -> TIS1_Distance [m]/1
  Abs/1 -> Trigonometric Function/1
  Trigonometric Function1/1 -> Product1/2
  Product1/1 -> Switch3/1
  TIS1 range max/1 -> Switch3/3
  Constant/1 -> Switch1/3
  Compare To Constant/1 -> Switch1/2, Switch3/2

== system ACC_Model/ACC_System/TIS1 Straight Road/TIS1 Sorting Fun ==
  note: === TIS1 Sorting Fun block ===
      |
      |  - transforms information from the first sensor
      |    to the more appropriate form.
  TIS1range [m] : Inport
  TIS1rangedot [m/s] : Inport  Port=2
  TIS1theta [deg] : Inport  Port=3
  Degrees to Radians : simulink_extras/Transformations/Degrees to Radians  SystemSampleTime=-1
  Switch : Switch  Criteria=u2 ~= 0
  Unary Minus : UnaryMinus
  Unary Minus1 : UnaryMinus
  range max : Constant  Value=TISMaxRange(1)
  TIS1_RANGE [m] : Outport
  TIS1_RANGEDOT [m/s] : Outport  Port=2
  TIS1_THETA [rad] : Outport  Port=3
  wires:
  Unary Minus/1 -> Degrees to Radians/1
  Switch/1 -> TIS1_RANGE [m]/1
  TIS1rangedot [m/s]/1 -> Unary Minus1/1
  range max/1 -> Switch/3
  Degrees to Radians/1 -> TIS1_THETA [rad]/1
  TIS1range [m]/1 -> Switch/2, Switch/1
  TIS1theta [deg]/1 -> Unary Minus/1
  Unary Minus1/1 -> TIS1_RANGEDOT [m/s]/1

== system ACC_Model/ACC_System/TIS2 ACC action/If Action Subsystem ==
  rd : Inport
  e : Inport  Port=2
  Vp : Inport  Port=3
  EGO distance : Inport  Port=4
  HWT dem : Inport  Port=5
  th in : Inport  Port=6
  Action Port : ActionPort  PropagateVarSize=During execution  ActionType=then
  If : If  IfExpression=u1 <= 0
  If Action Subsystem : Subsystem  TreatAsAtomicUnit=on
  If Action Subsystem1 : Subsystem  TreatAsAtomicUnit=on
  Merge : Merge
  Merge1 : Merge
  e1 : InportShadow  Port=2
  th in1 : InportShadow  Port=6
  dec : Outport  InitialOutput=0
  throttle : Outport  Port=2  InitialOutput=0
  wires:
  rd/1 -> If/1, If Action Subsystem1/1(rd)
  If/1 -> If Action Subsystem/Action
  If/2 -> If Action Subsystem1/Action
  e/1 -> If Action Subsystem/1(e)
  If Action Subsystem/1(brake) -> Merge/1
  If Action Subsystem1/1(dec) -> Merge/2
  If Action Subsystem/2(throttle) -> Merge1/1
  If Action Subsystem1/2(throttle) -> Merge1/2
  Merge/1 -> dec/1
  Merge1/1 -> throttle/1
  Vp/1 -> If Action Subsystem1/3(Vp)
  e1/1 -> If Action Subsystem1/2(e)
  EGO distance/1 -> If Action Subsystem1/4(EGO distance)
  HWT dem/1 -> If Action Subsystem1/5(HWT_dem)
  th in/1 -> If Action Subsystem/2(th_in)
  th in1/1 -> If Action Subsystem1/6(th_in)

== system ACC_Model/ACC_System/TIS2 ACC action/If Action Subsystem1 ==
  rd : Inport
  e : Inport  Port=2
  Vp : Inport  Port=3
  EGO dis : Inport  Port=4
  HWT dem : Inport  Port=5
  Action Port : ActionPort  PropagateVarSize=During execution  ActionType=else
  If : If  IfExpression=u1 <= 0
  If Action Subsystem : Subsystem  TreatAsAtomicUnit=on
  If Action Subsystem1 : Subsystem  TreatAsAtomicUnit=on
  Merge : Merge
  Merge1 : Merge
  dec : Outport  InitialOutput=0
  throttle : Outport  Port=2  InitialOutput=0
  wires:
  rd/1 -> If/1, If Action Subsystem1/1(rd)
  If/1 -> If Action Subsystem/Action
  If/2 -> If Action Subsystem1/Action
  Vp/1 -> If Action Subsystem1/3(Vp)
  If Action Subsystem/1(dec) -> Merge/1
  If Action Subsystem1/2(throttle) -> Merge1/2
  Merge/1 -> dec/1
  Merge1/1 -> throttle/1
  If Action Subsystem1/1(dec) -> Merge/2
  If Action Subsystem/2(throttle) -> Merge1/1
  e/1 -> If Action Subsystem1/2(e)
  EGO dis/1 -> If Action Subsystem1/4(Ego distance)
  HWT dem/1 -> If Action Subsystem1/5(HWT dem)

== system ACC_Model/ACC_System/TIS2 ACC action/Stop & Go ==
  Brake_Pres_in[bar] : Inport
  Throttle_in[%] : Inport  Port=2
  TIS2_Distance[m] : Inport  Port=3
  TIS2_HWT_flag : Inport  Port=4
  TIS2_Safe_Distance [m] : Inport  Port=5
  Vp [m/s] : Inport  Port=6
  Rangedot [m/s] : Inport  Port=7
  EGO_Velocity [m/s] : Inport  Port=8
  Stand : Inport  Port=9
  Gain : Gain  Gain=3.6
  If : If  IfExpression=u1 == 1
  If Action Subsystem : Subsystem  TreatAsAtomicUnit=on
  If Action Subsystem1 : Subsystem  TreatAsAtomicUnit=on
  Logical Operator : Logic  AllPortsSameDT=off  OutDataTypeStr=boolean
  LowActiv : Constant  Value=LowSpeedActv
  Merge : Merge
  Merge1 : Merge
  Rangedot [m/s]1 : InportShadow  Port=7
  Relational Operator1 : RelationalOperator  Operator=>  OutDataTypeStr=boolean
  Subsystem : Subsystem
  BrakePres[bar] : Outport
  Th_out [%] : Outport  Port=2
  wires:
  TIS2_Distance[m]/1 -> If Action Subsystem/1(TIS2_Distance[m])
  TIS2_Safe_Distance [m]/1 -> If Action Subsystem/2(TIS2_Safe_Distance [m])
  Vp [m/s]/1 -> Gain/1, If Action Subsystem/5(Vp)
  LowActiv/1 -> Relational Operator1/1
  Logical Operator/1 -> If/1
  Gain/1 -> Relational Operator1/2
  If/2 -> If Action Subsystem1/Action
  Throttle_in[%]/1 -> If Action Subsystem1/1(In1), If Action Subsystem/4(th_in)
  Brake_Pres_in[bar]/1 -> If Action Subsystem1/2(In2)
  Merge/1 -> Th_out [%]/1
  If Action Subsystem1/2(Out2) -> Merge1/2
  If/1 -> If Action Subsystem/Action
  If Action Subsystem1/1(Out1) -> Merge/2
  Rangedot [m/s]1/1 -> Subsystem/1(In1)
  Subsystem/1(BrakePres[bar]) -> BrakePres[bar]/1
  EGO_Velocity [m/s]/1 -> Subsystem/3(EGO_Velocity [m/s])
  Rangedot [m/s]/1 -> If Action Subsystem/3(rd)
  If Action Subsystem/1(br) -> Merge1/1
  If Action Subsystem/2(th) -> Merge/1
  TIS2_HWT_flag/1 -> Logical Operator/1
  Relational Operator1/1 -> Logical Operator/2
  Merge1/1 -> Subsystem/2(In2)
  Stand/1 -> If Action Subsystem/6(Stand)

== system ACC_Model/ACC_System/TIS2 Bend Road/Hold ==
  HWTflagIN : Inport
  lead_vel_in : Inport  Port=2
  HWTflagIN1 : InportShadow  Port=1
  If : If  IfExpression=u1 < 0.1  SampleTime=Tsensor
  If Action Subsystem : Subsystem  TreatAsAtomicUnit=on
  If Action Subsystem1 : Subsystem  TreatAsAtomicUnit=on
  Merge : Merge
  HWT_flag : Outport
  wires:
  lead_vel_in/1 -> If/1
  If/1 -> If Action Subsystem/Action
  If/2 -> If Action Subsystem1/Action
  If Action Subsystem/1(Out1) -> Merge/1
  If Action Subsystem1/1(Out1) -> Merge/2
  Merge/1 -> HWT_flag/1
  HWTflagIN/1 -> If Action Subsystem1/1(In1)
  HWTflagIN1/1 -> If Action Subsystem/1(In1)

== system ACC_Model/ACC_System/TIS2 Bend Road/Lead Car Longitudinal Velocity ==
  note: === TIS2 Lead Car Longitudinal Velocity block ===
      |
      |  - computes the leading car absolute velocity and safe distance between the EGO and leading car.
  HWT_dem (s) : Inport
  TIS1 Rangedot [m/s] : Inport  Port=2
  EGO Velocity [m/s] : Inport  Port=3
  Standstill [m] : Inport  Port=4
  theta [rad] : Inport  Port=5
  lambda [rad] : Inport  Port=6
  TIS2 Range [m] : Inport  Port=7
  Abs : Abs
  Add : Sum  Inputs=+-
  Add1 : Sum  Inputs=+-
  Constant : Constant  Value=0
  Divide : Product  Inputs=*/
  Divide2 : Product  Inputs=*/
  HWT_dem (s)1 : InportShadow  Port=1
  Product : Product  RndMeth=Zero
  Relational Operator : RelationalOperator  Operator=<=  OutDataTypeStr=boolean
  Switch : Switch  Criteria=u2 > Threshold
  Switch1 : Switch  Threshold=5*TISMaxRange(2)
  Trigonometric Function : Trigonometry  Operator=cos
  Safe distance [m] : Outport
  Lead velocity [m/s] : Outport  Port=2
  wires:
  Relational Operator/1 -> Switch/2
  Divide/1 -> Relational Operator/2
  HWT_dem (s)1/1 -> Divide/2
  Standstill [m]/1 -> Switch/1, Divide/1
  Switch/1 -> Safe distance [m]/1
  Product/1 -> Switch/3
  HWT_dem (s)/1 -> Product/2
  Add/1 -> Abs/1
  TIS1 Rangedot [m/s]/1 -> Divide2/1
  lambda [rad]/1 -> Add1/1
  theta [rad]/1 -> Add1/2
  Add1/1 -> Trigonometric Function/1
  Trigonometric Function/1 -> Divide2/2
  Divide2/1 -> Add/2
  EGO Velocity [m/s]/1 -> Add/1
  Abs/1 -> Product/1, Relational Operator/1, Switch1/3
  TIS2 Range [m]/1 -> Switch1/2
  Constant/1 -> Switch1/1
  Switch1/1 -> Lead velocity [m/s]/1

== system ACC_Model/ACC_System/TIS2 Bend Road/TIS1 HWT Computing ==
  note: === TIS1 HWT Computing block===
      |
      |  - computes HeadWay Time (HWT) as it is defined in ISO norms.
  Distance [m] : Inport
  Velocity [m/s] : Inport  Port=2
  If : If
  If Action Subsystem : Subsystem  TreatAsAtomicUnit=on
  If Action Subsystem1 : Subsystem  TreatAsAtomicUnit=on
  Merge : Merge
  HWT [s] : Outport
  wires:
  Velocity [m/s]/1 -> If/1, If Action Subsystem/2(Velocity [m/s])
  If/1 -> If Action Subsystem/Action
  If/2 -> If Action Subsystem1/Action
  If Action Subsystem/1(HWT [s]) -> Merge/1
  If Action Subsystem1/1(Out1) -> Merge/2
  Merge/1 -> HWT [s]/1
  Distance [m]/1 -> If Action Subsystem/1(Distance [m])

== system ACC_Model/ACC_System/TIS2 Bend Road/TIS2 Closest Object On Bend Road ==
  note: === TIS2 Closest Object block ===
      |
      |  - passing through data about potentially the most dangerous object driving on the bend road.
  index : Inport
  TIS2_range [m] : Inport  Port=2
  TIS2_rangedot [m] : Inport  Port=3
  TIS2_theta [rad] : Inport  Port=4
  TIS2_Distance [m] : Inport  Port=5
  TIS2_lambda [rad] : Inport  Port=6
  Constant2 : Constant  Value=5*TISMaxRange(2)
  Selector{1..3,6..7} (5 alike) : Selector  InputPortWidth=TISdet(2)  IndexOptions=Index vector (port)  Indices=[1 3]  OutputSizes=1
  Switch : Switch  Criteria=u2 ~= 0
  rangedot [m/s] : Outport
  theta [rad] : Outport  Port=2
  Distance [m] : Outport  Port=3
  range [m] : Outport  Port=4
  lambda [rad] : Outport  Port=5
  wires:
  TIS2_rangedot [m]/1 -> Selector2/1
  TIS2_range [m]/1 -> Selector1/1
  index/1 -> Selector1/2, Selector2/2, Selector3/2, Selector6/2, Selector7/2
  TIS2_theta [rad]/1 -> Selector3/1
  TIS2_Distance [m]/1 -> Selector6/1
  TIS2_lambda [rad]/1 -> Selector7/1
  Selector1/1 -> range [m]/1
  Selector2/1 -> rangedot [m/s]/1
  Selector3/1 -> theta [rad]/1
  Selector7/1 -> lambda [rad]/1
  Selector6/1 -> Switch/2, Switch/1
  Constant2/1 -> Switch/3
  Switch/1 -> Distance [m]/1

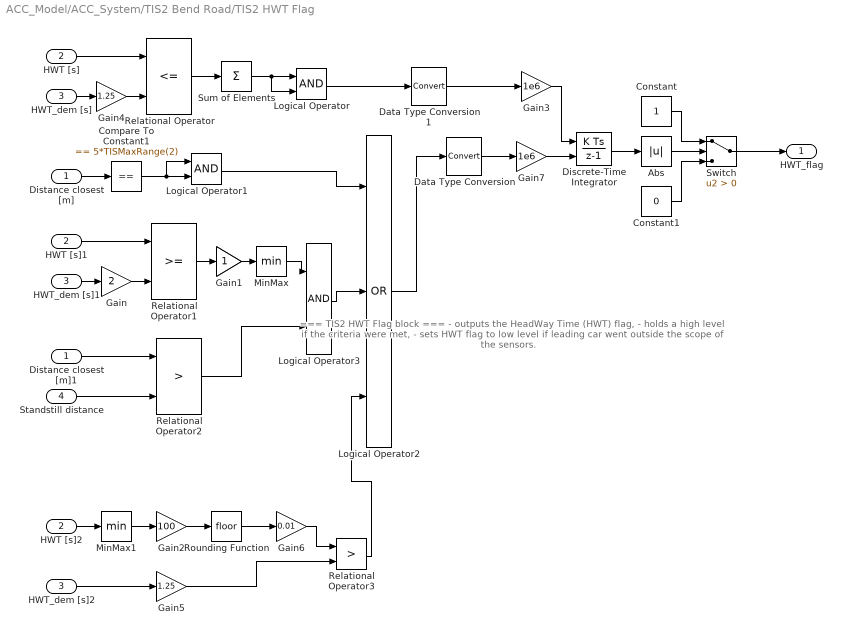
== system ACC_Model/ACC_System/TIS2 Bend Road/TIS2 HWT Flag ==
  note: === TIS2 HWT Flag block ===
      |
      |  - outputs the HeadWay Time (HWT) flag,
      |  - holds a high level if the criteria were met,
      |  - sets HWT flag to low level if leading car
      |    went outside the scope of the sensors.
  Distance closest [m] : Inport
  HWT [s] : Inport  Port=2
  HWT_dem [s] : Inport  Port=3
  Standstill distance : Inport  Port=4
  Abs : Abs
  Compare To Constant1 : simulink/Logic and Bit Operations/Compare To Constant  SystemSampleTime=-1  relop===  const=5*TISMaxRange(2)  LogicOutDataTypeMode=uint8
  Constant : Constant
  Constant1 : Constant  Value=0
  Data Type Conversion : DataTypeConversion
  Data Type Conversion1 : DataTypeConversion
  Discrete-Time Integrator : DiscreteIntegrator  ExternalReset=level  SampleTime=Tsensor  ICPrevOutput=DiscIntNeverNeededParam  ICPrevScaledInput=DiscIntNeverNeededParam
  Distance closest [m]1 : InportShadow  Port=1
  Gain : Gain  Gain=2
  Gain1 : Gain
  Gain2 : Gain  Gain=100
  Gain3 : Gain  Gain=1e6  OutDataTypeStr=double
  Gain4 : Gain  Gain=1.25
  Gain5 : Gain  Gain=1.25
  Gain6 : Gain  Gain=0.01
  Gain7 : Gain  Gain=1e6  OutDataTypeStr=double
  HWT [s]1 : InportShadow  Port=2
  HWT [s]2 : InportShadow  Port=2
  HWT_dem [s]1 : InportShadow  Port=3
  HWT_dem [s]2 : InportShadow  Port=3
  Logical Operator : Logic  AllPortsSameDT=off  OutDataTypeStr=boolean
  Logical Operator1 : Logic  AllPortsSameDT=off  OutDataTypeStr=boolean
  Logical Operator2 : Logic  Operator=OR  Inputs=3  AllPortsSameDT=off  OutDataTypeStr=boolean
  Logical Operator3 : Logic  AllPortsSameDT=off  OutDataTypeStr=boolean
  MinMax : MinMax
  MinMax1 : MinMax
  Relational Operator : RelationalOperator  Operator=<=  OutDataTypeStr=boolean
  Relational Operator1 : RelationalOperator  OutDataTypeStr=boolean
  Relational Operator2 : RelationalOperator  Operator=>  OutDataTypeStr=boolean
  Relational Operator3 : RelationalOperator  Operator=>  OutDataTypeStr=boolean
  Rounding Function : Rounding
  Sum of Elements : Sum  Inputs=+
  Switch : Switch  Criteria=u2 > Threshold
  HWT_flag : Outport
  wires:
  Logical Operator1/1 -> Logical Operator2/1
  Distance closest [m]/1 -> Compare To Constant1/1
  Logical Operator/1 -> Data Type Conversion1/1
  Sum of Elements/1 -> Logical Operator/2, Logical Operator/1
  Relational Operator/1 -> Sum of Elements/1
  HWT_dem [s]/1 -> Gain4/1
  HWT [s]/1 -> Relational Operator/1
  Compare To Constant1/1 -> Logical Operator1/2, Logical Operator1/1
  HWT [s]1/1 -> Relational Operator1/1
  Gain/1 -> Relational Operator1/2
  Relational Operator1/1 -> Gain1/1
  Gain1/1 -> MinMax/1
  HWT_dem [s]1/1 -> Gain/1
  Distance closest [m]1/1 -> Relational Operator2/1
  Standstill distance/1 -> Relational Operator2/2
  Relational Operator2/1 -> Logical Operator3/2
  MinMax/1 -> Logical Operator3/1
  Logical Operator3/1 -> Logical Operator2/2
  Gain3/1 -> Discrete-Time Integrator/1
  Switch/1 -> HWT_flag/1
  Abs/1 -> Switch/2
  Constant/1 -> Switch/1
  Constant1/1 -> Switch/3
  Discrete-Time Integrator/1 -> Abs/1
  Gain4/1 -> Relational Operator/2
  HWT_dem [s]2/1 -> Gain5/1
  HWT [s]2/1 -> MinMax1/1
  Logical Operator2/1 -> Data Type Conversion/1
  Gain2/1 -> Rounding Function/1
  Rounding Function/1 -> Gain6/1
  MinMax1/1 -> Gain2/1
  Gain6/1 -> Relational Operator3/1
  Gain5/1 -> Relational Operator3/2
  Relational Operator3/1 -> Logical Operator2/3
  Data Type Conversion/1 -> Gain7/1
  Data Type Conversion1/1 -> Gain3/1
  Gain7/1 -> Discrete-Time Integrator/2

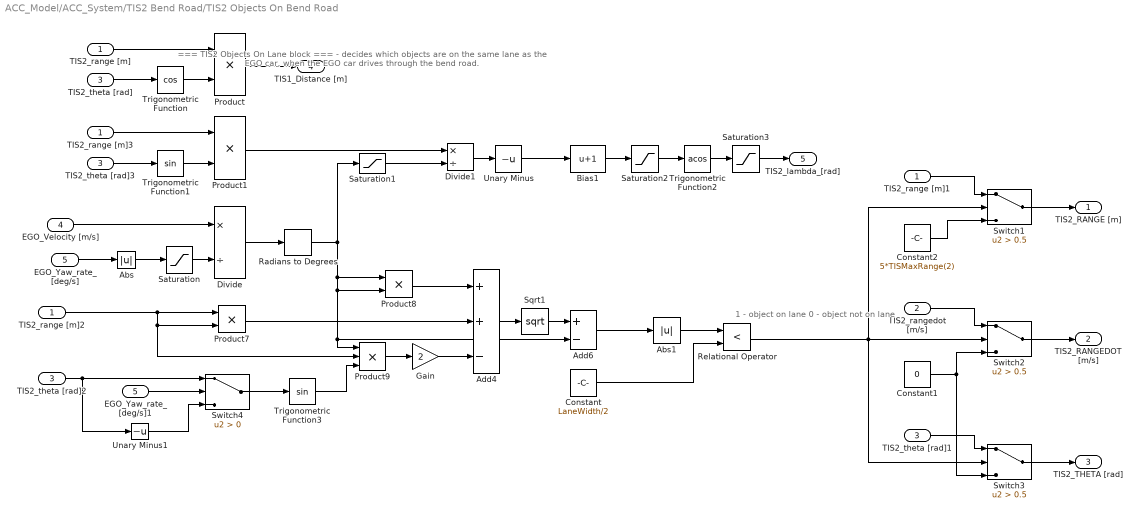
== system ACC_Model/ACC_System/TIS2 Bend Road/TIS2 Objects On Bend Road ==
  note: 1  - object      on lane
      | 0 - object not on lane
  note: === TIS2 Objects On Lane block ===
      |
      |  - decides which objects are on the same lane as the EGO car,
      |     when the EGO car drives through the bend road.
  TIS2_range [m] : Inport
  TIS2_rangedot [m/s] : Inport  Port=2
  TIS2_theta [rad] : Inport  Port=3
  EGO_Velocity [m/s] : Inport  Port=4
  EGO_Yaw_rate_[deg/s] : Inport  Port=5
  Abs : Abs
  Abs1 : Abs
  Add4 : Sum  Inputs=++-
  Add6 : Sum  Inputs=+-
  Bias1 : Bias  Bias=1
  Constant : Constant  Value=LaneWidth/2
  Constant1 : Constant  Value=0
  Constant2 : Constant  Value=5*TISMaxRange(2)
  Divide : Product  Inputs=*/
  Divide1 : Product  Inputs=*/
  EGO_Yaw_rate_[deg/s]1 : InportShadow  Port=5
  Gain : Gain  Gain=2
  Product{,1,7..8} (4 alike) : Product  RndMeth=Zero
  Product9 : Product  Inputs=3  RndMeth=Zero
  Radians to Degrees : simulink_extras/Transformations/Radians to Degrees  SystemSampleTime=-1
  Relational Operator : RelationalOperator  Operator=<  OutDataTypeStr=boolean
  Saturation : Saturate  UpperLimit=inf  LowerLimit=1e-6
  Saturation1 : Saturate  UpperLimit=inf  LowerLimit=1e-6
  Saturation2 : Saturate  UpperLimit=1  LowerLimit=-1
  Saturation3 : Saturate  UpperLimit=pi  LowerLimit=0
  Sqrt1 : Math  Operator=sqrt  SaturateOnIntegerOverflow=on
  Switch1 : Switch  Criteria=u2 > Threshold  Threshold=0.5
  Switch2 : Switch  Criteria=u2 > Threshold  Threshold=0.5
  Switch3 : Switch  Criteria=u2 > Threshold  Threshold=0.5
  Switch4 : Switch  Criteria=u2 > Threshold
  TIS2_range [m]1 : InportShadow  Port=1
  TIS2_range [m]2 : InportShadow  Port=1
  TIS2_range [m]3 : InportShadow  Port=1
  TIS2_theta [rad]1 : InportShadow  Port=3
  TIS2_theta [rad]2 : InportShadow  Port=3
  TIS2_theta [rad]3 : InportShadow  Port=3
  Trigonometric Function : Trigonometry  Operator=cos
  Trigonometric Function1 : Trigonometry
  Trigonometric Function2 : Trigonometry  Operator=acos
  Trigonometric Function3 : Trigonometry
  Unary Minus : UnaryMinus
  Unary Minus1 : UnaryMinus
  TIS2_RANGE [m] : Outport
  TIS2_RANGEDOT [m/s] : Outport  Port=2
  TIS2_THETA [rad] : Outport  Port=3
  TIS1_Distance [m] : Outport  Port=4
  TIS2_lambda_[rad] : Outport  Port=5
  wires:
  TIS2_range [m]/1 -> Product/1
  TIS2_theta [rad]/1 -> Trigonometric Function/1
  Trigonometric Function/1 -> Product/2
  Trigonometric Function1/1 -> Product1/2
  EGO_Velocity [m/s]/1 -> Divide/1
  EGO_Yaw_rate_[deg/s]/1 -> Abs/1
  Divide/1 -> Radians to Degrees/1
  Radians to Degrees/1 -> Product8/1, Product8/2, Product9/1, Add6/2, Saturation1/1
  Relational Operator/1 -> Switch1/2, Switch2/2, Switch3/2
  TIS2_rangedot [m/s]/1 -> Switch2/1
  TIS2_range [m]1/1 -> Switch1/1
  TIS2_theta [rad]1/1 -> Switch3/1
  Constant1/1 -> Switch2/3, Switch3/3
  Constant2/1 -> Switch1/3
  Switch1/1 -> TIS2_RANGE [m]/1
  Switch2/1 -> TIS2_RANGEDOT [m/s]/1
  Switch3/1 -> TIS2_THETA [rad]/1
  Bias1/1 -> Saturation2/1
  Divide1/1 -> Unary Minus/1
  Unary Minus/1 -> Bias1/1
  Trigonometric Function2/1 -> Saturation3/1
  Product/1 -> TIS1_Distance [m]/1
  Product8/1 -> Add4/1
  Product7/1 -> Add4/2
  Gain/1 -> Add4/3
  Product9/1 -> Gain/1
  Trigonometric Function3/1 -> Product9/3
  Add4/1 -> Sqrt1/1
  Sqrt1/1 -> Add6/1
  Add6/1 -> Abs1/1
  EGO_Yaw_rate_[deg/s]1/1 -> Switch4/2
  Switch4/1 -> Trigonometric Function3/1
  TIS2_theta [rad]2/1 -> Switch4/1, Unary Minus1/1
  Unary Minus1/1 -> Switch4/3
  TIS2_range [m]2/1 -> Product7/1, Product7/2, Product9/2
  TIS2_range [m]3/1 -> Product1/1
  TIS2_theta [rad]3/1 -> Trigonometric Function1/1
  Product1/1 -> Divide1/1
  Abs1/1 -> Relational Operator/1
  Constant/1 -> Relational Operator/2
  Saturation/1 -> Divide/2
  Saturation1/1 -> Divide1/2
  Saturation2/1 -> Trigonometric Function2/1
  Saturation3/1 -> TIS2_lambda_[rad]/1
  Abs/1 -> Saturation/1
